simulink subsystem "AccurateModel"  (R2024b)
settings: Solver=VariableStepAuto  StartTime=0.0  StopTime=10.0  RelTol=1e-3
settings Model: Creator=federico  LastModifiedBy=federico

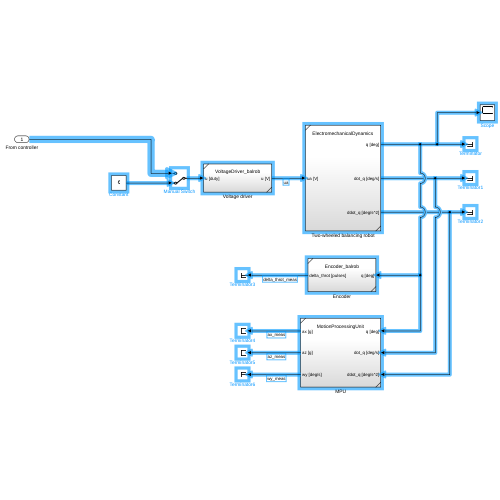
[thumbnail: Simulink's stored preview of the top-level diagram]
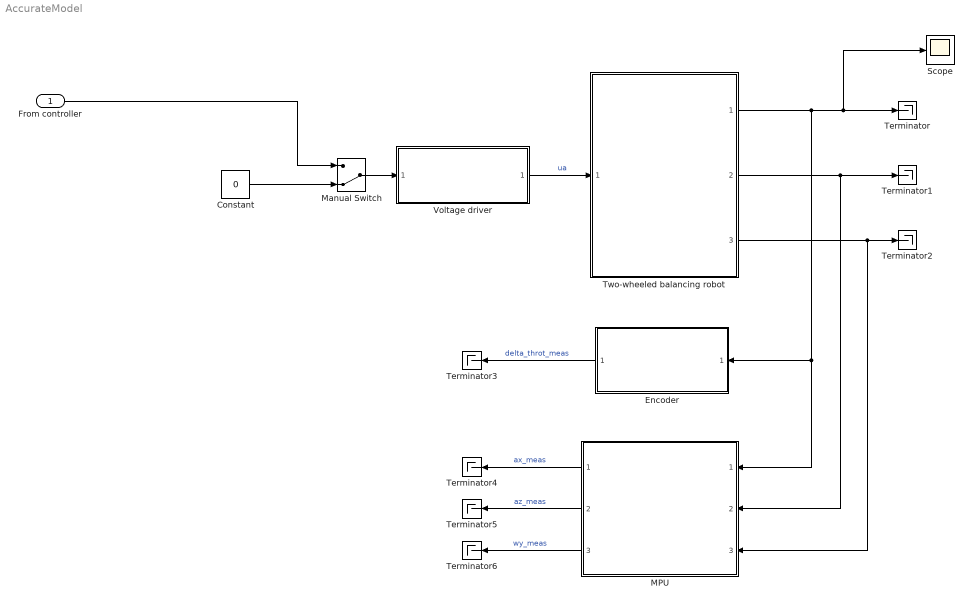
== system AccurateModel ==
  From controller : Inport
  Constant : Constant  Value=0
  Encoder : Subsystem  ReferencedSubsystem=Encoder_balrob
  MPU : Subsystem  ReferencedSubsystem=MotionProcessingUnit
  Manual Switch : ManualSwitch  CurrentSetting=0
  Scope : Scope
  Terminator{,1..6} (7 alike) : Terminator
  Two-wheeled balancing robot : Subsystem  ReferencedSubsystem=ElectromechanicalDynamics
  Voltage driver : Subsystem  ReferencedSubsystem=VoltageDriver_balrob
  wires:
  Voltage driver/1 -> Two-wheeled balancing robot/1  "ua"
  Two-wheeled balancing robot/2 -> Terminator1/1, MPU/2
  Two-wheeled balancing robot/3 -> MPU/3, Terminator2/1
  Encoder/1 -> Terminator3/1  "delta_throt_meas"
  MPU/1 -> Terminator4/1  "ax_meas"
  MPU/2 -> Terminator5/1  "az_meas"
  MPU/3 -> Terminator6/1  "wy_meas"
  Manual Switch/1 -> Voltage driver/1
  Constant/1 -> Manual Switch/2
  From controller/1 -> Manual Switch/1
  Two-wheeled balancing robot/1 -> MPU/1, Encoder/1, Terminator/1, Scope/1
